simulink model "interpolationEx"  (R2015a)
settings: Solver=ode45  StartTime=0.0  StopTime=1  RelTol=1e-3
values from neighbouring files (symbols this model uses):
  xdata_1 = [0:0.1:10]    [run_InterpolationEx.m]
  xdata_2 = [0:0.1:10]    [run_InterpolationEx.m]
  xdata_3 = [0:0.1:10]    [run_InterpolationEx.m]
  xint_1 = 5    [run_InterpolationEx.m]
  xint_2 = 5    [run_InterpolationEx.m]
  xint_3 = 4    [run_InterpolationEx.m]
  ydata_1 = sin(xdata_1) + 0.5*xdata_1    [run_InterpolationEx.m]
  ydata_2 = [0:0.1:10]    [run_InterpolationEx.m]
  ydata_3 = [0:0.1:10]    [run_InterpolationEx.m]
  yint_2 = 8    [run_InterpolationEx.m]
  yint_3 = 5    [run_InterpolationEx.m]
  zdata_3 = [0:0.1:10]    [run_InterpolationEx.m]
  zint_3 = zdata_3(ind)    [run_InterpolationEx.m]
undefined symbols (not defined in the file or in its folder): vdata_3, zdata_2
libraries: lib_GenTools_1DlinearInterp x1, lib_GenTools_2DlinearInterp x1, lib_GenTools_3DlinearInterp x1
settings Model: Creator=jlkratz  LastModifiedBy=jlkratz

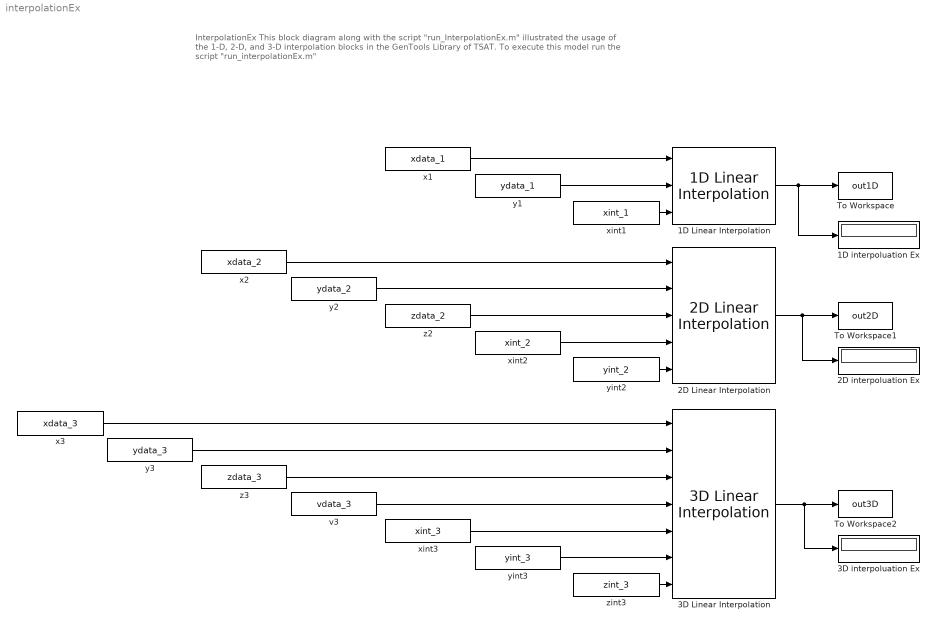
== system interpolationEx ==
  note: InterpolationEx
      |
      | This block diagram along with the script "run_InterpolationEx.m" illustrated the usage of the 1-D, 2-D, and 3-D interpolation
      | blocks in the GenTools Library of TSAT.
      |
      | To execute this model run the script "run_interpolationEx.m"
  1D Linear Interpolation : lib_GenTools_1DlinearInterp/1D Linear Interpolation  BN_M=double(gcb)
  1D interpoluation Ex : Display
  2D Linear Interpolation : lib_GenTools_2DlinearInterp/2D Linear Interpolation  BN_M=double(gcb)
  2D interpoluation Ex : Display
  3D Linear Interpolation : lib_GenTools_3DlinearInterp/3D Linear Interpolation  BN_M=double(gcb)
  3D interpoluation Ex : Display
  To Workspace : ToWorkspace  VariableName=out1D  SaveFormat=Timeseries  SampleTime=-1
      settings: MaxDataPoints=1
  To Workspace1 : ToWorkspace  VariableName=out2D  SaveFormat=Timeseries  SampleTime=-1
      settings: MaxDataPoints=1
  To Workspace2 : ToWorkspace  VariableName=out3D  SaveFormat=Timeseries  SampleTime=-1
      settings: MaxDataPoints=1
  v3 : Constant  Value=vdata_3
  x1 : Constant  Value=xdata_1
  x2 : Constant  Value=xdata_2
  x3 : Constant  Value=xdata_3
  xint1 : Constant  Value=xint_1
  xint2 : Constant  Value=xint_2
  xint3 : Constant  Value=xint_3
  y1 : Constant  Value=ydata_1
  y2 : Constant  Value=ydata_2
  y3 : Constant  Value=ydata_3
  yint2 : Constant  Value=yint_2
  yint3 : Constant  Value=yint_3
  z2 : Constant  Value=zdata_2
  z3 : Constant  Value=zdata_3
  zint3 : Constant  Value=zint_3
  wires:
  1D Linear Interpolation/1 -> 1D interpoluation Ex/1, To Workspace/1
  2D Linear Interpolation/1 -> 2D interpoluation Ex/1, To Workspace1/1
  3D Linear Interpolation/1 -> 3D interpoluation Ex/1, To Workspace2/1
  x1/1 -> 1D Linear Interpolation/1
  y1/1 -> 1D Linear Interpolation/2
  xint1/1 -> 1D Linear Interpolation/3
  x2/1 -> 2D Linear Interpolation/1
  y2/1 -> 2D Linear Interpolation/2
  yint2/1 -> 2D Linear Interpolation/5
  z2/1 -> 2D Linear Interpolation/3
  xint2/1 -> 2D Linear Interpolation/4
  xint3/1 -> 3D Linear Interpolation/5
  zint3/1 -> 3D Linear Interpolation/7
  yint3/1 -> 3D Linear Interpolation/6
  x3/1 -> 3D Linear Interpolation/1
  y3/1 -> 3D Linear Interpolation/2
  z3/1 -> 3D Linear Interpolation/3
  v3/1 -> 3D Linear Interpolation/4
